simulink subsystem "lazo_control_corriente"  (R2023b)
settings: Solver=VariableStepAuto  StartTime=0.0  StopTime=10.0  RelTol=1e-3
values from neighbouring files (symbols this model uses):
  R_0 = 4    [parametros.m]
  R_d = 33    [parametros.m]
  R_q = 29    [parametros.m]
settings Model: Creator=nicol  LastModifiedBy=nicol

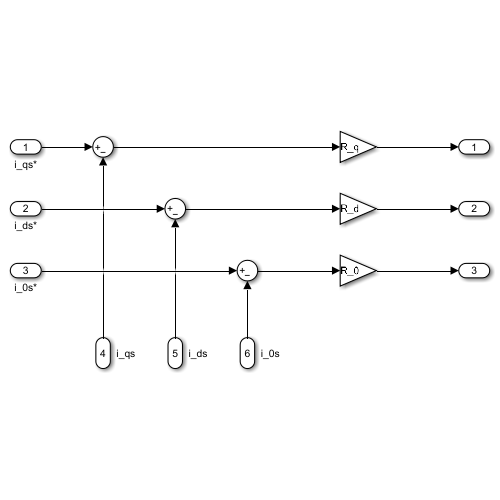
[thumbnail: Simulink's stored preview of the top-level diagram]
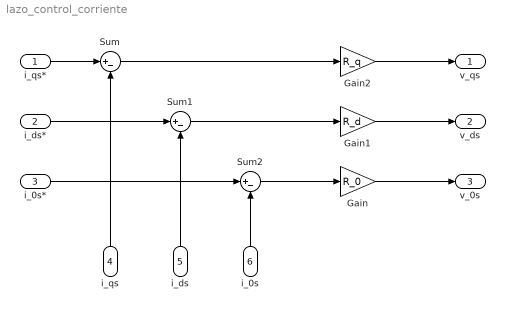
== system lazo_control_corriente ==
  i_qs* : Inport
  i_ds* : Inport  Port=2
  i_0s* : Inport  Port=3
  i_qs : Inport  Port=4
  i_ds : Inport  Port=5
  i_0s : Inport  Port=6
  Gain : Gain  Gain=R_0
  Gain1 : Gain  Gain=R_d
  Gain2 : Gain  Gain=R_q
  Sum : Sum  Inputs=|+-
  Sum1 : Sum  Inputs=|+-
  Sum2 : Sum  Inputs=|+-
  v_qs : Outport
  v_ds : Outport  Port=2
  v_0s : Outport  Port=3
  wires:
  Sum/1 -> Gain2/1
  Sum2/1 -> Gain/1
  Sum1/1 -> Gain1/1
  Gain/1 -> v_0s/1
  Gain1/1 -> v_ds/1
  Gain2/1 -> v_qs/1
  i_qs*/1 -> Sum/1
  i_ds*/1 -> Sum1/1
  i_0s*/1 -> Sum2/1
  i_qs/1 -> Sum/2
  i_ds/1 -> Sum1/2
  i_0s/1 -> Sum2/2
